simulink model "Sine_HDL"  (R2023a)
settings: Solver=VariableStepAuto  StartTime=0.0  StopTime=1  RelTol=1e-3
undefined symbols (not defined in the file): S, vsva5601, xcvp2502
libraries: hdlBasic x2, vmcUtilities x1
settings Model: Creator=sdegala  LastModifiedBy=sdegala

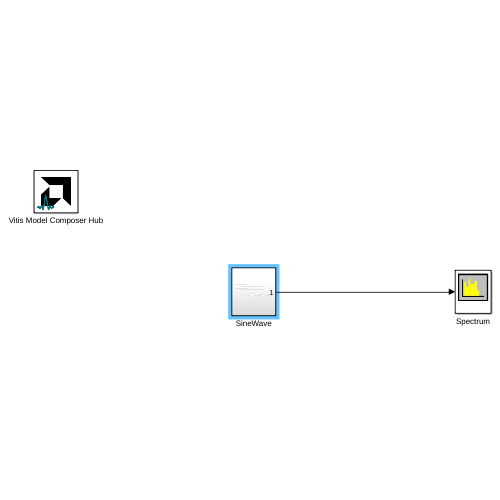
[thumbnail: Simulink's stored preview of the top-level diagram]
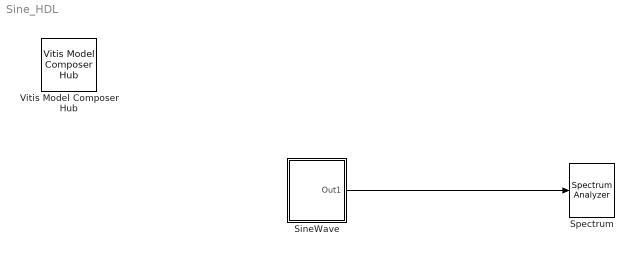
== system Sine_HDL ==
  SineWave : Subsystem
  Spectrum : SpectrumAnalyzer  WindowPosition=[1.000000,41.000000,1280.000000,600.000000,]  Visible=on  ScopeFrameLocation=window  SampleRate=100000  Span=50000  StartFrequency=-50000  StopFrequency=50000  AveragingMethod=Exponential  YLimits=[-85.09147716,36.09192634]  ShowLegend=on
  Vitis Model Composer Hub : vmcUtilities/Vitis Model Composer Hub  Tag=genX  CodeGeneration=off  SubsystemName=SineWave  CompilationType=HDLCompilation  ExportTypeV2=IP Catalog  TargetDirectory=./netlist  exportDesign=off  analyzeDesign=off  validateDesignOnHw=off  ExportType=AI Engines  IpVendor=xilinx.com  IpLibrary=hls  IpVersion=1.0  IpHWLanguage=Verilog  AieCompilerOptions={}  AieSimulatorOptions={}  CreateTestbench=off  TestbenchStackSize=10  RunRtlSim=off  RunCSim=off  RunAieSim=off  AieSimTimeout=50000  RunAieSimProfiling=off  LaunchVitisAnalyzer=off  PlotOutput=off  RunX86Sim=off  X86SimTimeout=10  GenHwImage=off  GenLibadfXo=on  GenHwValidationCode=off  PlatformType=Not Specified  HwSystemType=Baremetal  HwValidationTarget=hw  ProjDevice=xcvp2502-vsva5601-1LP-e-S  ProjDevicePart=xcvp2502-vsva5601-1LP-e-S  AIEType=AIE  SamplePeriod=-1  ClockFrequency=200  DataPathParallelism=1  xilinxfamily=versalpremium  part=xcvp2502  speed=-1LP-e-S  package=vsva5601  directory=./netlist/ip/SineWave/src  testbench=off  incr_netlist=off  synthesis_tool=Vivado  clock_wrapper=Clock Enables  dbl_ovrd=According to Block Masks  dcm_input_clock_period=10  sysclk_period=10  simulink_period=1/100e6  eval_field=0  LogFileName=''  NThreads=4
  wires:
  SineWave/1(Out1) -> Spectrum/1

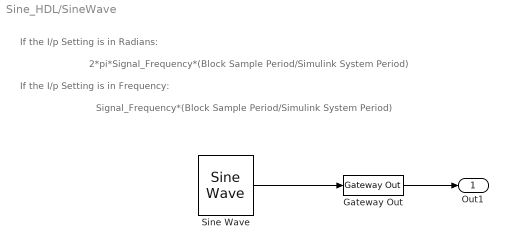
== system Sine_HDL/SineWave ==
  note: Signal_Frequency*(Block Sample Period/Simulink System Period)
  note: If the I/p Setting is in Frequency:
  note: If the I/p Setting is in Radians:
  note: 2*pi*Signal_Frequency*(Block Sample Period/Simulink System Period)
  Gateway Out : hdlBasic/Gateway Out  inherit_from_input=on  hdl_port=on  rows=1  columns=1  UseAsDAC=off  DACChannel='1'  interface=None  automatic_assignment=on  address_offset=hex2dec('00')  intf_name=''  intf_description=''  timing_constraint=None  locs_specified=off  LOCs={}  io_standard={}  XmcBlockStatus=1  maskContainerNames=group4  block_type=gatewayout  block_config=sysgen:gateway_out_config  block_width_w=590  block_height_w=620  block_width=620  block_height=750
  Sine Wave : hdlBasic/Sine Wave  Input_format=Frequency  output_frequency=5e6  phase_offset_angles=0  output_selection=Sine  sfdr=90  explicit_period=off  period=1  simulation_type=fast_sim  simulation_model=sysgen:dds_macro  XmcBlockStatus=1  maskContainerNames=oportetch  block_type=dds_macro  block_config=sysgen:DDSMacro_config
  Out1 : Outport
  wires:
  Sine Wave/1 -> Gateway Out/1
  Gateway Out/1 -> Out1/1
